simulink model "UDEF_PLL"  (R2023b)
settings: Solver=VariableStepAuto  StartTime=0.0  StopTime=30  RelTol=1e-3
undefined symbols (not defined in the file or in its folder): DiscIntNeverNeededParam, f_test, Fbase, fpll, k_lpf, lpf_A, lpf_B, lpf_C, lpf_D, Ts, wc_lpf
libraries: SimplusGT x4
settings Model: Creator=yz34218  LastModifiedBy=yz34218

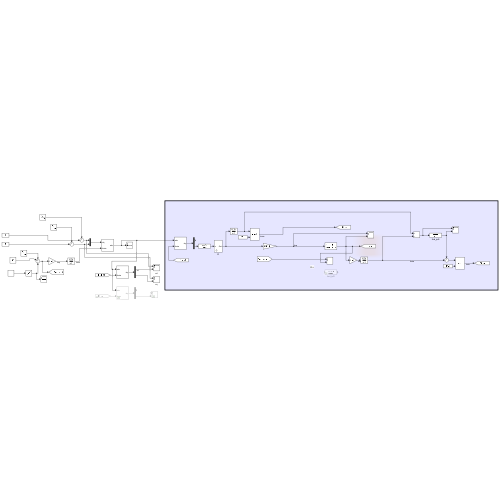
[thumbnail: Simulink's stored preview of the top-level diagram]
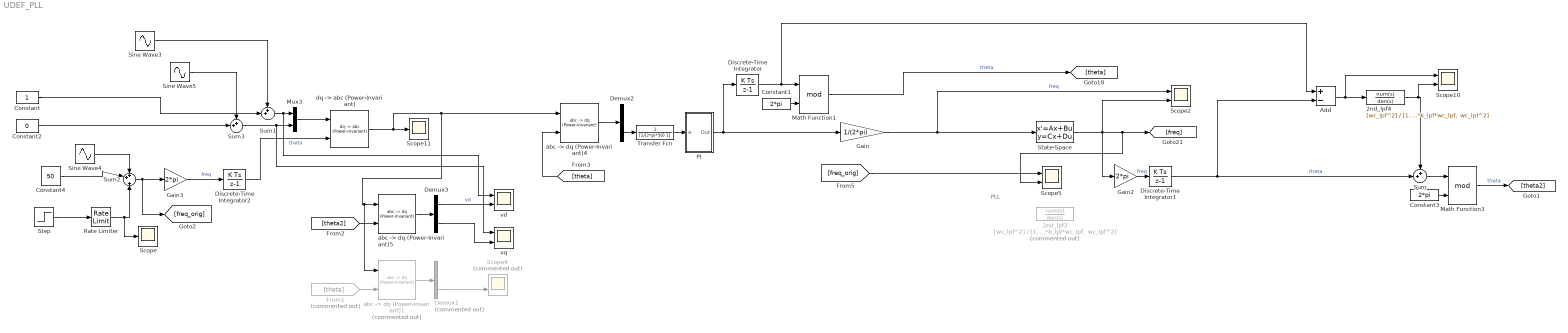
== system UDEF_PLL ==
  note: PLL
  2nd_lpf2 : TransferFcn  Commented=on  Numerator=[wc_lpf^2]  Denominator="[1, 2*k_lpf*wc_lpf,  wc_lpf^2]"
  2nd_lpf4 : TransferFcn  Numerator=[wc_lpf^2]  Denominator="[1, 2*k_lpf*wc_lpf,  wc_lpf^2]"
  Add : Sum  Inputs=+-
  Constant : Constant
  Constant1 : Constant  Value=2*pi
  Constant2 : Constant  Value=0
  Constant3 : Constant  Value=2*pi
  Constant4 : Constant  Value=50
  Demux1 : Demux  Commented=on  Outputs=2
  Demux2 : Demux  Outputs=2
  Demux3 : Demux  Outputs=2
  Discrete-Time Integrator : DiscreteIntegrator  SampleTime=Ts  ICPrevOutput=DiscIntNeverNeededParam  ICPrevScaledInput=DiscIntNeverNeededParam
  Discrete-Time Integrator1 : DiscreteIntegrator  SampleTime=Ts  ICPrevOutput=DiscIntNeverNeededParam  ICPrevScaledInput=DiscIntNeverNeededParam
  Discrete-Time Integrator2 : DiscreteIntegrator  SampleTime=Ts  ICPrevOutput=DiscIntNeverNeededParam  ICPrevScaledInput=DiscIntNeverNeededParam
  From1 : From  Commented=on  GotoTag=theta
  Gain : Gain  Gain=1/(2*pi)
  Gain2 : Gain  Gain=2*pi
  Gain3 : Gain  Gain=2*pi
  Math Function1 : Math  Operator=mod  SignedPower=on
  Math Function3 : Math  Operator=mod  SignedPower=on
  Mux3 : Mux  Inputs=2
  PI : Subsystem  mask{Kp_PLL=2*pi*fpll, Ki_PLL=(2*pi*fpll)^2/4, IntSat_PLL=20000}
      mask prompts: Kp_PLL "Proportional (P)"; Ki_PLL "Integral (I)"; IntSat_PLL "Integrator Saturation Limit"
      mask DialogControl DescGroupVar Prompt: PLL Parameters
  Rate Limiter : RateLimiter  RisingSlewLimit=0.2/10  FallingSlewLimit=-0.2/10  SampleTimeMode=inherited
  Scope : Scope
  Scope10 : Scope  NumInputPorts=2
  Scope11 : Scope
  Scope2 : Scope  NumInputPorts=2
  Scope4 : Scope  Commented=on  NumInputPorts=2
  Scope5 : Scope  NumInputPorts=2
  Sine Wave3 : Sin  Amplitude=0.3  Frequency=2*pi*f_test  SampleTime=0
  Sine Wave4 : Sin  Amplitude=0  Frequency=2*pi*f_test  SampleTime=0
  Sine Wave5 : Sin  Amplitude=0.3  Frequency=2*pi*f_test  SampleTime=0
  State-Space : StateSpace  A=lpf_A  B=lpf_B  C=lpf_C  D=lpf_D  InitialCondition=[0,50/lpf_C(2)]
  Step : Step  After=0.2  SampleTime=0
  Sum : Sum  Inputs=++|
  Sum1 : Sum  Inputs=++|
  Sum2 : Sum  Inputs=++|+
  Sum3 : Sum  Inputs=++|
  Transfer Fcn : TransferFcn  Denominator=[1/(2*pi*50) 1]
  "abc -> dq (Power-Invariant)1" : SimplusGT/abc -> dq (Power-Invariant)  Commented=on  SystemSampleTime=-1  VariantActivationTime=update diagram  AllowFlexibleInterface=on  Latency=0  AutoFrameSizeCalculation=off
      settings: SourceProductName=Simplus Grid Tool
  "abc -> dq (Power-Invariant)4" : SimplusGT/abc -> dq (Power-Invariant)  SystemSampleTime=-1  VariantActivationTime=update diagram  AllowFlexibleInterface=on  Latency=0  AutoFrameSizeCalculation=off
      settings: SourceProductName=Simplus Grid Tool
  "abc -> dq (Power-Invariant)5" : SimplusGT/abc -> dq (Power-Invariant)  SystemSampleTime=-1  VariantActivationTime=update diagram  AllowFlexibleInterface=on  Latency=0  AutoFrameSizeCalculation=off
      settings: SourceProductName=Simplus Grid Tool
  "dq -> abc (Power-Invariant)" : SimplusGT/dq -> abc (Power-Invariant)  SystemSampleTime=-1  VariantActivationTime=update diagram  AllowFlexibleInterface=on  Latency=0  AutoFrameSizeCalculation=off
      settings: SourceProductName=Simplus Grid Tool
  vd : Scope  NumInputPorts=2
  vq : Scope  NumInputPorts=2
  wires:
  2nd_lpf4/1 -> Sum/1, Scope10/2
  State-Space/1 -> Scope5/2, [freq], Scope2/2, Gain2/1
  Math Function3/1 -> [theta2]  "theta"
  Constant3/1 -> Math Function3/2
  Sum/1 -> Math Function3/1
  Gain2/1 -> Discrete-Time Integrator1/1  "freq"
  Discrete-Time Integrator/1 -> Math Function1/1, Add/1
  Constant1/1 -> Math Function1/2
  Add/1 -> 2nd_lpf4/1, Scope10/1
  Transfer Fcn/1 -> PI/1(e)
  Math Function1/1 -> [theta]  "theta"
  Gain/1 -> State-Space/1, Scope2/1  "freq"
  PI/1(Out) -> Gain/1, Discrete-Time Integrator/1
  Discrete-Time Integrator1/1 -> Add/2, Sum/2  "theta"
  Mux3/1 -> "dq -> abc (Power-Invariant)"/1
  Constant/1 -> Sum1/2
  Sum1/1 -> vd/1, Mux3/1
  Sine Wave3/1 -> Sum1/1
  Gain3/1 -> Discrete-Time Integrator2/1  "freq"
  Discrete-Time Integrator2/1 -> "dq -> abc (Power-Invariant)"/2  "theta"
  "dq -> abc (Power-Invariant)"/1 -> "abc -> dq (Power-Invariant)1"/1, "abc -> dq (Power-Invariant)5"/1, "abc -> dq (Power-Invariant)4"/1, Scope11/1
  "abc -> dq (Power-Invariant)4"/1 -> Demux2/1
  Demux2/2 -> Transfer Fcn/1
  [theta] -> "abc -> dq (Power-Invariant)4"/2
  [theta2] -> "abc -> dq (Power-Invariant)5"/2
  "abc -> dq (Power-Invariant)5"/1 -> Demux3/1
  Constant4/1 -> Sum2/2
  Sum2/1 -> [freq_orig], Gain3/1
  Sine Wave4/1 -> Sum2/1
  [freq_orig] -> Scope5/1
  Step/1 -> Rate Limiter/1
  Rate Limiter/1 -> Scope/1, Sum2/3
  Demux3/1 -> vd/2  "vd"
  Demux3/2 -> vq/2
  From1/1 -> "abc -> dq (Power-Invariant)1"/2
  "abc -> dq (Power-Invariant)1"/1 -> Demux1/1
  Demux1/2 -> Scope4/2
  Constant2/1 -> Sum3/2
  Sum3/1 -> vq/1, Mux3/2
  Sine Wave5/1 -> Sum3/1

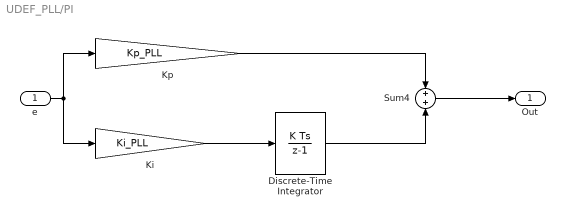
== system UDEF_PLL/PI ==
  e : Inport
  Discrete-Time Integrator : DiscreteIntegrator  gainval=1  InitialCondition=2*pi*Fbase  SampleTime=Ts  LimitOutput=on  UpperSaturationLimit=2*pi*Fbase + IntSat_PLL  LowerSaturationLimit=2*pi*Fbase - IntSat_PLL  ICPrevOutput=DiscIntNeverNeededParam  ICPrevScaledInput=DiscIntNeverNeededParam
  Ki : Gain  Gain=Ki_PLL  SaturateOnIntegerOverflow=on  OutDataTypeStr=Inherit: Same as input  ParamDataTypeStr=Inherit: Same as input
  Kp : Gain  Gain=Kp_PLL  SaturateOnIntegerOverflow=on  OutDataTypeStr=Inherit: Same as input  ParamDataTypeStr=Inherit: Same as input
  Sum4 : Sum  SaturateOnIntegerOverflow=on
  Out : Outport
  wires:
  Ki/1 -> Discrete-Time Integrator/1
  Kp/1 -> Sum4/1
  e/1 -> Ki/1, Kp/1
  Discrete-Time Integrator/1 -> Sum4/2
  Sum4/1 -> Out/1
